simulink model "visual_aid1"  (R2021b)
settings: Solver=VariableStepAuto  StartTime=0.0  StopTime=10.0  RelTol=1e-3
libraries: dspsrcs4 x2
settings Model: Creator=kschutz  LastModifiedBy=kschutz

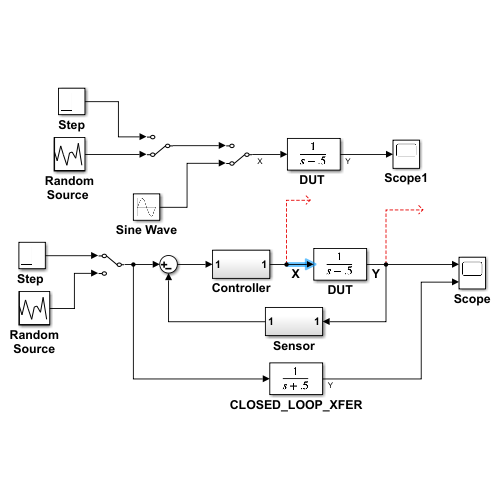
[thumbnail: Simulink's stored preview of the top-level diagram]
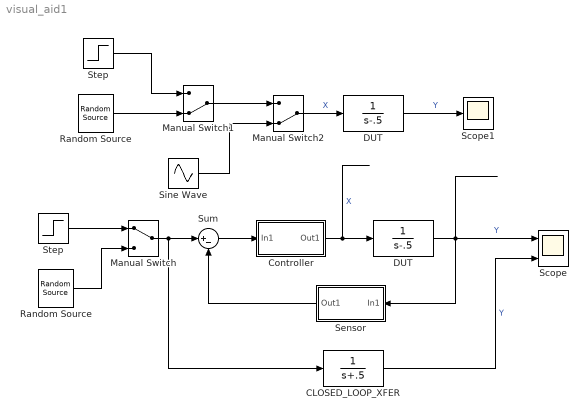
== system visual_aid1 ==
  CLOSED_LOOP_XFER : TransferFcn  Denominator=[1 .5]
  Controller : Subsystem
  DUT : TransferFcn  Denominator=[1 -.5]
  "DUT " : TransferFcn  Denominator=[1 -.5]
  Manual Switch : ManualSwitch
  Manual Switch1 : ManualSwitch  CurrentSetting=0
  Manual Switch2 : ManualSwitch  CurrentSetting=0
  Random Source : dspsrcs4/Random Source  SrcType=Uniform  NormMethod=Ziggurat  CltLength=12  MinVal=0  MaxVal=1  MeanVal=0  VarVal=1  RepMode=Not repeatable  rawSeed=1  IsInherit=off  SampMode=Discrete  SampTime=1  SampFrame=1  DataType=Double  OutComplex=Real  OutputFrames=off
  "Random Source " : dspsrcs4/Random Source  SrcType=Uniform  NormMethod=Ziggurat  CltLength=12  MinVal=0  MaxVal=1  MeanVal=0  VarVal=1  RepMode=Not repeatable  rawSeed=1  IsInherit=off  SampMode=Discrete  SampTime=1  SampFrame=1  DataType=Double  OutComplex=Real  OutputFrames=off
  Scope : Scope  NumInputPorts=2
  Scope1 : Scope
  Sensor : Subsystem
  Sine Wave : Sin  Frequency=2*pi*1  SampleTime=0
  Step : Step  SampleTime=0
  "Step " : Step  SampleTime=0
  Sum : Sum  Inputs=|+-
  wires:
  Sum/1 -> Controller/1(In1)
  DUT/1 -> Scope/1, Sensor/1(In1)  "Y"
  Controller/1(Out1) -> DUT/1  "X"
  "DUT "/1 -> Scope1/1  "Y"
  "Step "/1 -> Manual Switch/1
  Random Source/1 -> Manual Switch/2
  Manual Switch/1 -> CLOSED_LOOP_XFER/1, Sum/1
  Step/1 -> Manual Switch1/1
  "Random Source "/1 -> Manual Switch1/2
  Manual Switch2/1 -> "DUT "/1  "X"
  Manual Switch1/1 -> Manual Switch2/1
  Sine Wave/1 -> Manual Switch2/2
  Sensor/1(Out1) -> Sum/2
  CLOSED_LOOP_XFER/1 -> Scope/2  "Y"

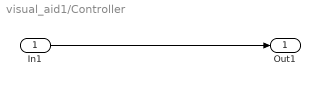
== system visual_aid1/Controller ==
  In1 : Inport
  Out1 : Outport
  wires:
  In1/1 -> Out1/1

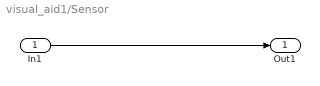
== system visual_aid1/Sensor ==
  In1 : Inport
  Out1 : Outport
  wires:
  In1/1 -> Out1/1
